simulink model "ExponentialHornDiscretized_frequencyResponse"  (Simulink 7.8)
settings: Solver=FixedStepDiscrete  StartTime=0.0  StopTime=1.0  FixedStep=1.0  RelTol=1e-3
undefined symbols (not defined in the file): areaChange, simpleDuct
settings Model: Creator=emmert  LastModifiedBy=smith

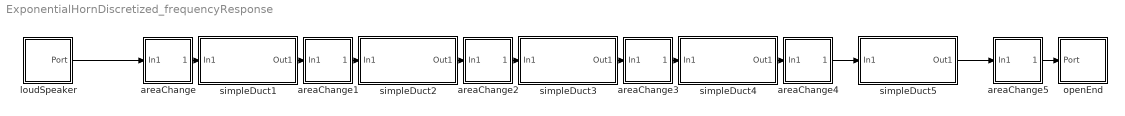
== system ExponentialHornDiscretized_frequencyResponse ==
  areaChange : Subsystem  mask{aj=1.2214}
      mask prompts: aj "Area @Out1 (m²)"
      settings: AttributesFormatString=%<aj> m^2
      mask Display:
      | plot([-.5 1.1],[.5 .5])
      | 
      | patch([ .4  .4  .3  .3  .35 .35 .15 .1 .40 .40 .10 .15 .35 .60 .60 .75 .60 .60 .75 .65 .65 .6   .6 ], ...
      |       [-.05 .05 .05 .15 .2  .25 .3 .35 .35 .65 .65 .70 .75 .75 .65 .65 .55 .45 .35 .35 .05 .05 -.05], [.85 .85 .85])
      | plot([.40 .40 .10 .15 .35 .60 .60 .75 .60 .60], ...
      |      [.35 .65 .65 .70 .75 .75 .65 .65 .55 .40])
      | plot([.1  .45 .45 .3  .3  .35 .35 .15 .1 ], ...
      |      [.35 .35 .05 .05 .15 .2  .25 .3  .35])
      | plot([.55 .6  .6  .75 .65 .65 .55 .55], ...
      |      [.35 .35 .45 .35 .35 .05 .05 .35])
      | plot([.4   .4   .6  .6 ], ...
      |      [.05 -.2 -.2   .05])
      | plot([.4   .4   .6  .6 ], ...
      |      [.05 -.2 -.2   .05])
      | 
      | text(.8,.85,'A','HorizontalAlignment','center')
  areaChange1 : Subsystem  mask{aj=1.8221}
      mask prompts: aj "Area @Out1 (m²)"
      settings: AttributesFormatString=%<aj> m^2
      mask Display:
      | plot([-.5 1.1],[.5 .5])
      | 
      | patch([ .4  .4  .3  .3  .35 .35 .15 .1 .40 .40 .10 .15 .35 .60 .60 .75 .60 .60 .75 .65 .65 .6   .6 ], ...
      |       [-.05 .05 .05 .15 .2  .25 .3 .35 .35 .65 .65 .70 .75 .75 .65 .65 .55 .45 .35 .35 .05 .05 -.05], [.85 .85 .85])
      | plot([.40 .40 .10 .15 .35 .60 .60 .75 .60 .60], ...
      |      [.35 .65 .65 .70 .75 .75 .65 .65 .55 .40])
      | plot([.1  .45 .45 .3  .3  .35 .35 .15 .1 ], ...
      |      [.35 .35 .05 .05 .15 .2  .25 .3  .35])
      | plot([.55 .6  .6  .75 .65 .65 .55 .55], ...
      |      [.35 .35 .45 .35 .35 .05 .05 .35])
      | plot([.4   .4   .6  .6 ], ...
      |      [.05 -.2 -.2   .05])
      | plot([.4   .4   .6  .6 ], ...
      |      [.05 -.2 -.2   .05])
      | 
      | text(.8,.85,'A','HorizontalAlignment','center')
  areaChange2 : Subsystem  mask{aj=2.7183}
      mask prompts: aj "Area @Out1 (m²)"
      settings: AttributesFormatString=%<aj> m^2
      mask Display:
      | plot([-.5 1.1],[.5 .5])
      | 
      | patch([ .4  .4  .3  .3  .35 .35 .15 .1 .40 .40 .10 .15 .35 .60 .60 .75 .60 .60 .75 .65 .65 .6   .6 ], ...
      |       [-.05 .05 .05 .15 .2  .25 .3 .35 .35 .65 .65 .70 .75 .75 .65 .65 .55 .45 .35 .35 .05 .05 -.05], [.85 .85 .85])
      | plot([.40 .40 .10 .15 .35 .60 .60 .75 .60 .60], ...
      |      [.35 .65 .65 .70 .75 .75 .65 .65 .55 .40])
      | plot([.1  .45 .45 .3  .3  .35 .35 .15 .1 ], ...
      |      [.35 .35 .05 .05 .15 .2  .25 .3  .35])
      | plot([.55 .6  .6  .75 .65 .65 .55 .55], ...
      |      [.35 .35 .45 .35 .35 .05 .05 .35])
      | plot([.4   .4   .6  .6 ], ...
      |      [.05 -.2 -.2   .05])
      | plot([.4   .4   .6  .6 ], ...
      |      [.05 -.2 -.2   .05])
      | 
      | text(.8,.85,'A','HorizontalAlignment','center')
  areaChange3 : Subsystem  mask{aj=4.0552}
      mask prompts: aj "Area @Out1 (m²)"
      settings: AttributesFormatString=%<aj> m^2
      mask Display:
      | plot([-.5 1.1],[.5 .5])
      | 
      | patch([ .4  .4  .3  .3  .35 .35 .15 .1 .40 .40 .10 .15 .35 .60 .60 .75 .60 .60 .75 .65 .65 .6   .6 ], ...
      |       [-.05 .05 .05 .15 .2  .25 .3 .35 .35 .65 .65 .70 .75 .75 .65 .65 .55 .45 .35 .35 .05 .05 -.05], [.85 .85 .85])
      | plot([.40 .40 .10 .15 .35 .60 .60 .75 .60 .60], ...
      |      [.35 .65 .65 .70 .75 .75 .65 .65 .55 .40])
      | plot([.1  .45 .45 .3  .3  .35 .35 .15 .1 ], ...
      |      [.35 .35 .05 .05 .15 .2  .25 .3  .35])
      | plot([.55 .6  .6  .75 .65 .65 .55 .55], ...
      |      [.35 .35 .45 .35 .35 .05 .05 .35])
      | plot([.4   .4   .6  .6 ], ...
      |      [.05 -.2 -.2   .05])
      | plot([.4   .4   .6  .6 ], ...
      |      [.05 -.2 -.2   .05])
      | 
      | text(.8,.85,'A','HorizontalAlignment','center')
  areaChange4 : Subsystem  mask{aj=6.0496}
      mask prompts: aj "Area @Out1 (m²)"
      settings: AttributesFormatString=%<aj> m^2
      mask Display:
      | plot([-.5 1.1],[.5 .5])
      | 
      | patch([ .4  .4  .3  .3  .35 .35 .15 .1 .40 .40 .10 .15 .35 .60 .60 .75 .60 .60 .75 .65 .65 .6   .6 ], ...
      |       [-.05 .05 .05 .15 .2  .25 .3 .35 .35 .65 .65 .70 .75 .75 .65 .65 .55 .45 .35 .35 .05 .05 -.05], [.85 .85 .85])
      | plot([.40 .40 .10 .15 .35 .60 .60 .75 .60 .60], ...
      |      [.35 .65 .65 .70 .75 .75 .65 .65 .55 .40])
      | plot([.1  .45 .45 .3  .3  .35 .35 .15 .1 ], ...
      |      [.35 .35 .05 .05 .15 .2  .25 .3  .35])
      | plot([.55 .6  .6  .75 .65 .65 .55 .55], ...
      |      [.35 .35 .45 .35 .35 .05 .05 .35])
      | plot([.4   .4   .6  .6 ], ...
      |      [.05 -.2 -.2   .05])
      | plot([.4   .4   .6  .6 ], ...
      |      [.05 -.2 -.2   .05])
      | 
      | text(.8,.85,'A','HorizontalAlignment','center')
  areaChange5 : Subsystem  mask{aj=7.3891}
      mask prompts: aj "Area @Out1 (m²)"
      settings: AttributesFormatString=%<aj> m^2
      mask Display:
      | plot([-.5 1.1],[.5 .5])
      | 
      | patch([ .4  .4  .3  .3  .35 .35 .15 .1 .40 .40 .10 .15 .35 .60 .60 .75 .60 .60 .75 .65 .65 .6   .6 ], ...
      |       [-.05 .05 .05 .15 .2  .25 .3 .35 .35 .65 .65 .70 .75 .75 .65 .65 .55 .45 .35 .35 .05 .05 -.05], [.85 .85 .85])
      | plot([.40 .40 .10 .15 .35 .60 .60 .75 .60 .60], ...
      |      [.35 .65 .65 .70 .75 .75 .65 .65 .55 .40])
      | plot([.1  .45 .45 .3  .3  .35 .35 .15 .1 ], ...
      |      [.35 .35 .05 .05 .15 .2  .25 .3  .35])
      | plot([.55 .6  .6  .75 .65 .65 .55 .55], ...
      |      [.35 .35 .45 .35 .35 .05 .05 .35])
      | plot([.4   .4   .6  .6 ], ...
      |      [.05 -.2 -.2   .05])
      | plot([.4   .4   .6  .6 ], ...
      |      [.05 -.2 -.2   .05])
      | 
      | text(.8,.85,'A','HorizontalAlignment','center')
  loudSpeaker : Subsystem  mask{loc=Upstream, Amp=1, c=100, Mach=0, rho=1.2, D=2*sqrt(1/pi), element=loudSpeaker}
      mask prompts: loc "Location"; Amp "Foringamplitude [m/s]"; c "Speed of sound (m/s)"; Mach "Mach number (dimensionless)"; rho "Density (Kg/m³)"; D "Diameter (m)"
      mask init:
      | if Mach<0
      |    errordlg('Mach Number must be bigger than or equal to zero','invalid Mach Number');
      | end
      | 
      | 
      | if c<=0
      |     errordlg('speed of sound must be positive','invalid speed of sound');
      | end
      | 
      | 
      | if D<=0
      |      errordlg('diameter must be positive','invalid diameter');
      | 
      | end
      | 
      | 
      | if rho<=0
      |      errordlg('density must be positive','invalid density');
      | end
      | 
      | % Set identifier
      | set_param(gcb,'element',char('loudSpeaker'));
      | 
      | switchBCUpDownStream(gcb,loc);
      mask StyleString: popup(Downstream|Upstream),edit,edit,edit,edit,edit,edit
      mask Display:
      | plot([.2 .2 .4 .4 .2],[.6 .4 .4 .6 .6])
      | plot([.7 .7 .4 .4 .7],[.9 .1 .3 .7 .9])
  openEnd : Subsystem  mask{loc=Downstream, c=343, Mach=0.1, rho=1.2, D=1, element=openEnd}
      mask prompts: loc "Location"; c "Speed of sound (m/s)"; Mach "Mach number (dimensionless)"; rho "Density (Kg/m³)"; D "Diameter (m)"
      mask init:
      | if Mach<0
      |    errordlg('Mach Number must be bigger than or equal to zero','invalid Mach Number');
      | end
      | 
      | 
      | if c<=0
      |     errordlg('speed of sound must be positive','invalid speed of sound');
      | end
      | 
      | 
      | if D<=0
      |      errordlg('diameter must be positive','invalid diameter');
      | 
      | end
      | 
      | 
      | if rho<=0
      |      errordlg('density must be positive','invalid density');
      | end
      | 
      | % Set identifier
      | set_param(gcb,'element',char('openEnd'));
      | 
      | switchBCUpDownStream(gcb,loc);
      mask StyleString: popup(Downstream|Upstream),edit,edit,edit,edit,edit
      mask Display:
      | patch([.2  1  1 .2],[.2 .2 .8 .8],[.7 1 1])
      | patch([.2 .3 .3 .2],[.2 .2 .8 .8],[.9 1 1])
      | patch([.3 .4 .4 .3],[.2 .2 .8 .8],[.8 1 1])
      | plot([.3 1],[.2 .2])
      | plot([.3 1],[.8 .8])
      | plot([1 1 0 0 1],[1 0 0 1 1])
  simpleDuct1 : Subsystem  mask{l=0.2, damping_model_popup=no damping, gm=1.4, nu=1.568e-5, Pr=0.707, damping_model_id=1}
      mask prompts: l "Length [m]"; damping_model_popup "Damping model"; gm "Ratio of specific heats [-]"; nu "Kinematic Viscosity [m^2/s]"; Pr "Prandtl number [-]"; damping_model_id "damping"
      settings: AttributesFormatString=%<l> m
      mask StyleString: edit,popup(no damping|Kirchhoff (wide tubes)|Peters|Dokumanci (best but slow)|Howe (turbulent)),edit,edit,edit,edit
      mask CallbackString:
      | |% Get the mask parameter values. This is a cell
      | %   array of strings.
      | maskStr = get_param(gcb,'MaskValues');
      | 
      | % The pop-up menu is the first mask parameter.
      | %   Check pop-up choice by comparing first letter, i.e. n or K...
      | if strcmp(maskStr{2}(1),'n'),
      |     % Turn off visibility of gamma/nu/Pr
      |     set_param(gcb,'MaskVisibilities',{'on';'on';'off';'off';'off';'off'}),
      | 	maskStr{6} = '1';
      |     set_param(gcb,'MaskValues',maskStr);
      | elseif strcmp(maskStr{2}(1),'K'),
      | 	% turn on visibility of gamma/nu/Pr
      |     set_param(gcb,'MaskVisibilities',{'on';'on';'on';'on';'on';'off'}),
      | 	maskStr{6} = '2';
      |     set_param(gcb,'MaskValues',maskStr);
      | elseif strcmp(maskStr{2}(1),'P'),
      | 	% turn on visibility of gamma/nu/Pr
      |     set_param(gcb,'MaskVisibilities',{'on';'on';'on';'on';'on';'off'}),
      | 	maskStr{6} = '3';
      |     set_param(gcb,'MaskValues',maskStr);
      | elseif strcmp(maskStr{2}(1),'D'),
      | 	% turn on visibility of gamma/nu/Pr
      |     set_param(gcb,'MaskVisibilities',{'on';'on';'on';'on';'on';'off'}),
      | 	maskStr{6} = '4';
      |     set_param(gcb,'MaskValues',maskStr);
      | else
      | 	% turn on visibility of gamma/nu
      |     set_param(gcb,'MaskVisibilities',{'on';'on';'on';'on';'off';'off'}),
      | 	maskStr{6} = '5';
      |     set_param(gcb,'MaskValues',maskStr);
      | end||||
      mask Display:
      | patch([0 1 1 0],[.2 .2 .8 .8],[.7 1 1])
      | plot([0 1],[.2 .2])
      | plot([0 1],[.8 .8])
      | 
      | plot([1 1 0 0 1],[1 0 0 1 1])
  simpleDuct2 : Subsystem  mask{l=0.2, damping_model_popup=no damping, gm=1.4, nu=1.568e-5, Pr=0.707, damping_model_id=1}
      mask prompts: l "Length [m]"; damping_model_popup "Damping model"; gm "Ratio of specific heats [-]"; nu "Kinematic Viscosity [m^2/s]"; Pr "Prandtl number [-]"; damping_model_id "damping"
      settings: AttributesFormatString=%<l> m
      mask StyleString: edit,popup(no damping|Kirchhoff (wide tubes)|Peters|Dokumanci (best but slow)|Howe (turbulent)),edit,edit,edit,edit
      mask CallbackString:
      | |% Get the mask parameter values. This is a cell
      | %   array of strings.
      | maskStr = get_param(gcb,'MaskValues');
      | 
      | % The pop-up menu is the first mask parameter.
      | %   Check pop-up choice by comparing first letter, i.e. n or K...
      | if strcmp(maskStr{2}(1),'n'),
      |     % Turn off visibility of gamma/nu/Pr
      |     set_param(gcb,'MaskVisibilities',{'on';'on';'off';'off';'off';'off'}),
      | 	maskStr{6} = '1';
      |     set_param(gcb,'MaskValues',maskStr);
      | elseif strcmp(maskStr{2}(1),'K'),
      | 	% turn on visibility of gamma/nu/Pr
      |     set_param(gcb,'MaskVisibilities',{'on';'on';'on';'on';'on';'off'}),
      | 	maskStr{6} = '2';
      |     set_param(gcb,'MaskValues',maskStr);
      | elseif strcmp(maskStr{2}(1),'P'),
      | 	% turn on visibility of gamma/nu/Pr
      |     set_param(gcb,'MaskVisibilities',{'on';'on';'on';'on';'on';'off'}),
      | 	maskStr{6} = '3';
      |     set_param(gcb,'MaskValues',maskStr);
      | elseif strcmp(maskStr{2}(1),'D'),
      | 	% turn on visibility of gamma/nu/Pr
      |     set_param(gcb,'MaskVisibilities',{'on';'on';'on';'on';'on';'off'}),
      | 	maskStr{6} = '4';
      |     set_param(gcb,'MaskValues',maskStr);
      | else
      | 	% turn on visibility of gamma/nu
      |     set_param(gcb,'MaskVisibilities',{'on';'on';'on';'on';'off';'off'}),
      | 	maskStr{6} = '5';
      |     set_param(gcb,'MaskValues',maskStr);
      | end||||
      mask Display:
      | patch([0 1 1 0],[.2 .2 .8 .8],[.7 1 1])
      | plot([0 1],[.2 .2])
      | plot([0 1],[.8 .8])
      | 
      | plot([1 1 0 0 1],[1 0 0 1 1])
  simpleDuct3 : Subsystem  mask{l=0.2, damping_model_popup=no damping, gm=1.4, nu=1.568e-5, Pr=0.707, damping_model_id=1}
      mask prompts: l "Length [m]"; damping_model_popup "Damping model"; gm "Ratio of specific heats [-]"; nu "Kinematic Viscosity [m^2/s]"; Pr "Prandtl number [-]"; damping_model_id "damping"
      settings: AttributesFormatString=%<l> m
      mask StyleString: edit,popup(no damping|Kirchhoff (wide tubes)|Peters|Dokumanci (best but slow)|Howe (turbulent)),edit,edit,edit,edit
      mask CallbackString:
      | |% Get the mask parameter values. This is a cell
      | %   array of strings.
      | maskStr = get_param(gcb,'MaskValues');
      | 
      | % The pop-up menu is the first mask parameter.
      | %   Check pop-up choice by comparing first letter, i.e. n or K...
      | if strcmp(maskStr{2}(1),'n'),
      |     % Turn off visibility of gamma/nu/Pr
      |     set_param(gcb,'MaskVisibilities',{'on';'on';'off';'off';'off';'off'}),
      | 	maskStr{6} = '1';
      |     set_param(gcb,'MaskValues',maskStr);
      | elseif strcmp(maskStr{2}(1),'K'),
      | 	% turn on visibility of gamma/nu/Pr
      |     set_param(gcb,'MaskVisibilities',{'on';'on';'on';'on';'on';'off'}),
      | 	maskStr{6} = '2';
      |     set_param(gcb,'MaskValues',maskStr);
      | elseif strcmp(maskStr{2}(1),'P'),
      | 	% turn on visibility of gamma/nu/Pr
      |     set_param(gcb,'MaskVisibilities',{'on';'on';'on';'on';'on';'off'}),
      | 	maskStr{6} = '3';
      |     set_param(gcb,'MaskValues',maskStr);
      | elseif strcmp(maskStr{2}(1),'D'),
      | 	% turn on visibility of gamma/nu/Pr
      |     set_param(gcb,'MaskVisibilities',{'on';'on';'on';'on';'on';'off'}),
      | 	maskStr{6} = '4';
      |     set_param(gcb,'MaskValues',maskStr);
      | else
      | 	% turn on visibility of gamma/nu
      |     set_param(gcb,'MaskVisibilities',{'on';'on';'on';'on';'off';'off'}),
      | 	maskStr{6} = '5';
      |     set_param(gcb,'MaskValues',maskStr);
      | end||||
      mask Display:
      | patch([0 1 1 0],[.2 .2 .8 .8],[.7 1 1])
      | plot([0 1],[.2 .2])
      | plot([0 1],[.8 .8])
      | 
      | plot([1 1 0 0 1],[1 0 0 1 1])
  simpleDuct4 : Subsystem  mask{l=0.2, damping_model_popup=no damping, gm=1.4, nu=1.568e-5, Pr=0.707, damping_model_id=1}
      mask prompts: l "Length [m]"; damping_model_popup "Damping model"; gm "Ratio of specific heats [-]"; nu "Kinematic Viscosity [m^2/s]"; Pr "Prandtl number [-]"; damping_model_id "damping"
      settings: AttributesFormatString=%<l> m
      mask StyleString: edit,popup(no damping|Kirchhoff (wide tubes)|Peters|Dokumanci (best but slow)|Howe (turbulent)),edit,edit,edit,edit
      mask CallbackString:
      | |% Get the mask parameter values. This is a cell
      | %   array of strings.
      | maskStr = get_param(gcb,'MaskValues');
      | 
      | % The pop-up menu is the first mask parameter.
      | %   Check pop-up choice by comparing first letter, i.e. n or K...
      | if strcmp(maskStr{2}(1),'n'),
      |     % Turn off visibility of gamma/nu/Pr
      |     set_param(gcb,'MaskVisibilities',{'on';'on';'off';'off';'off';'off'}),
      | 	maskStr{6} = '1';
      |     set_param(gcb,'MaskValues',maskStr);
      | elseif strcmp(maskStr{2}(1),'K'),
      | 	% turn on visibility of gamma/nu/Pr
      |     set_param(gcb,'MaskVisibilities',{'on';'on';'on';'on';'on';'off'}),
      | 	maskStr{6} = '2';
      |     set_param(gcb,'MaskValues',maskStr);
      | elseif strcmp(maskStr{2}(1),'P'),
      | 	% turn on visibility of gamma/nu/Pr
      |     set_param(gcb,'MaskVisibilities',{'on';'on';'on';'on';'on';'off'}),
      | 	maskStr{6} = '3';
      |     set_param(gcb,'MaskValues',maskStr);
      | elseif strcmp(maskStr{2}(1),'D'),
      | 	% turn on visibility of gamma/nu/Pr
      |     set_param(gcb,'MaskVisibilities',{'on';'on';'on';'on';'on';'off'}),
      | 	maskStr{6} = '4';
      |     set_param(gcb,'MaskValues',maskStr);
      | else
      | 	% turn on visibility of gamma/nu
      |     set_param(gcb,'MaskVisibilities',{'on';'on';'on';'on';'off';'off'}),
      | 	maskStr{6} = '5';
      |     set_param(gcb,'MaskValues',maskStr);
      | end||||
      mask Display:
      | patch([0 1 1 0],[.2 .2 .8 .8],[.7 1 1])
      | plot([0 1],[.2 .2])
      | plot([0 1],[.8 .8])
      | 
      | plot([1 1 0 0 1],[1 0 0 1 1])
  simpleDuct5 : Subsystem  mask{l=0.2, damping_model_popup=no damping, gm=1.4, nu=1.568e-5, Pr=0.707, damping_model_id=1}
      mask prompts: l "Length [m]"; damping_model_popup "Damping model"; gm "Ratio of specific heats [-]"; nu "Kinematic Viscosity [m^2/s]"; Pr "Prandtl number [-]"; damping_model_id "damping"
      settings: AttributesFormatString=%<l> m
      mask StyleString: edit,popup(no damping|Kirchhoff (wide tubes)|Peters|Dokumanci (best but slow)|Howe (turbulent)),edit,edit,edit,edit
      mask CallbackString:
      | |% Get the mask parameter values. This is a cell
      | %   array of strings.
      | maskStr = get_param(gcb,'MaskValues');
      | 
      | % The pop-up menu is the first mask parameter.
      | %   Check pop-up choice by comparing first letter, i.e. n or K...
      | if strcmp(maskStr{2}(1),'n'),
      |     % Turn off visibility of gamma/nu/Pr
      |     set_param(gcb,'MaskVisibilities',{'on';'on';'off';'off';'off';'off'}),
      | 	maskStr{6} = '1';
      |     set_param(gcb,'MaskValues',maskStr);
      | elseif strcmp(maskStr{2}(1),'K'),
      | 	% turn on visibility of gamma/nu/Pr
      |     set_param(gcb,'MaskVisibilities',{'on';'on';'on';'on';'on';'off'}),
      | 	maskStr{6} = '2';
      |     set_param(gcb,'MaskValues',maskStr);
      | elseif strcmp(maskStr{2}(1),'P'),
      | 	% turn on visibility of gamma/nu/Pr
      |     set_param(gcb,'MaskVisibilities',{'on';'on';'on';'on';'on';'off'}),
      | 	maskStr{6} = '3';
      |     set_param(gcb,'MaskValues',maskStr);
      | elseif strcmp(maskStr{2}(1),'D'),
      | 	% turn on visibility of gamma/nu/Pr
      |     set_param(gcb,'MaskVisibilities',{'on';'on';'on';'on';'on';'off'}),
      | 	maskStr{6} = '4';
      |     set_param(gcb,'MaskValues',maskStr);
      | else
      | 	% turn on visibility of gamma/nu
      |     set_param(gcb,'MaskVisibilities',{'on';'on';'on';'on';'off';'off'}),
      | 	maskStr{6} = '5';
      |     set_param(gcb,'MaskValues',maskStr);
      | end||||
      mask Display:
      | patch([0 1 1 0],[.2 .2 .8 .8],[.7 1 1])
      | plot([0 1],[.2 .2])
      | plot([0 1],[.8 .8])
      | 
      | plot([1 1 0 0 1],[1 0 0 1 1])
  wires:
  loudSpeaker/1(Port) -> areaChange/1(In1)
  areaChange/1(Out1) -> simpleDuct1/1(In1)
  simpleDuct1/1(Out1) -> areaChange1/1(In1)
  areaChange1/1(Out1) -> simpleDuct2/1(In1)
  simpleDuct2/1(Out1) -> areaChange2/1(In1)
  areaChange2/1(Out1) -> simpleDuct3/1(In1)
  simpleDuct3/1(Out1) -> areaChange3/1(In1)
  areaChange3/1(Out1) -> simpleDuct4/1(In1)
  simpleDuct4/1(Out1) -> areaChange4/1(In1)
  areaChange4/1(Out1) -> simpleDuct5/1(In1)
  simpleDuct5/1(Out1) -> areaChange5/1(In1)
  areaChange5/1(Out1) -> openEnd/1(Port)

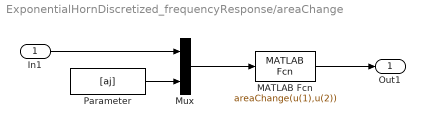
== system ExponentialHornDiscretized_frequencyResponse/areaChange ==
  In1 : Inport
  MATLAB Fcn : MATLABFcn  MATLABFcn=areaChange(u(1),u(2))  OutputDimensions=1  OutputSignalType=real
  Mux : Mux  Inputs=2
  Parameter : Constant  Value=[aj]
  Out1 : Outport
  wires:
  Parameter/1 -> Mux/2
  Mux/1 -> MATLAB Fcn/1
  MATLAB Fcn/1 -> Out1/1
  In1/1 -> Mux/1

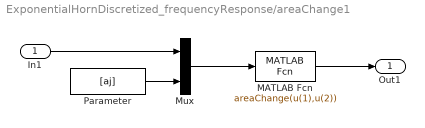
== system ExponentialHornDiscretized_frequencyResponse/areaChange1 ==
  In1 : Inport
  MATLAB Fcn : MATLABFcn  MATLABFcn=areaChange(u(1),u(2))  OutputDimensions=1  OutputSignalType=real
  Mux : Mux  Inputs=2
  Parameter : Constant  Value=[aj]
  Out1 : Outport
  wires:
  Parameter/1 -> Mux/2
  Mux/1 -> MATLAB Fcn/1
  MATLAB Fcn/1 -> Out1/1
  In1/1 -> Mux/1

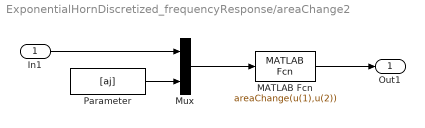
== system ExponentialHornDiscretized_frequencyResponse/areaChange2 ==
  In1 : Inport
  MATLAB Fcn : MATLABFcn  MATLABFcn=areaChange(u(1),u(2))  OutputDimensions=1  OutputSignalType=real
  Mux : Mux  Inputs=2
  Parameter : Constant  Value=[aj]
  Out1 : Outport
  wires:
  Parameter/1 -> Mux/2
  Mux/1 -> MATLAB Fcn/1
  MATLAB Fcn/1 -> Out1/1
  In1/1 -> Mux/1

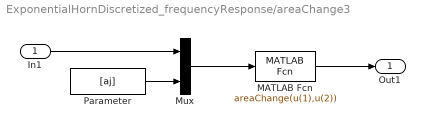
== system ExponentialHornDiscretized_frequencyResponse/areaChange3 ==
  In1 : Inport
  MATLAB Fcn : MATLABFcn  MATLABFcn=areaChange(u(1),u(2))  OutputDimensions=1  OutputSignalType=real
  Mux : Mux  Inputs=2
  Parameter : Constant  Value=[aj]
  Out1 : Outport
  wires:
  Parameter/1 -> Mux/2
  Mux/1 -> MATLAB Fcn/1
  MATLAB Fcn/1 -> Out1/1
  In1/1 -> Mux/1

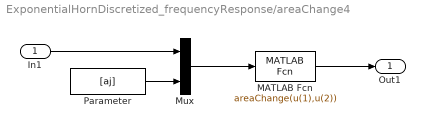
== system ExponentialHornDiscretized_frequencyResponse/areaChange4 ==
  In1 : Inport
  MATLAB Fcn : MATLABFcn  MATLABFcn=areaChange(u(1),u(2))  OutputDimensions=1  OutputSignalType=real
  Mux : Mux  Inputs=2
  Parameter : Constant  Value=[aj]
  Out1 : Outport
  wires:
  Parameter/1 -> Mux/2
  Mux/1 -> MATLAB Fcn/1
  MATLAB Fcn/1 -> Out1/1
  In1/1 -> Mux/1

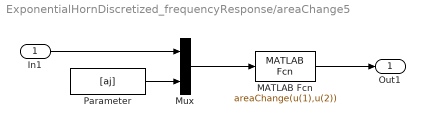
== system ExponentialHornDiscretized_frequencyResponse/areaChange5 ==
  In1 : Inport
  MATLAB Fcn : MATLABFcn  MATLABFcn=areaChange(u(1),u(2))  OutputDimensions=1  OutputSignalType=real
  Mux : Mux  Inputs=2
  Parameter : Constant  Value=[aj]
  Out1 : Outport
  wires:
  Parameter/1 -> Mux/2
  Mux/1 -> MATLAB Fcn/1
  MATLAB Fcn/1 -> Out1/1
  In1/1 -> Mux/1

== system ExponentialHornDiscretized_frequencyResponse/loudSpeaker ==
  Port : Outport

== system ExponentialHornDiscretized_frequencyResponse/openEnd ==
  Port : Inport

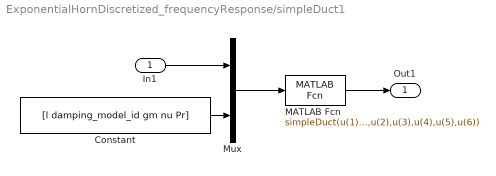
== system ExponentialHornDiscretized_frequencyResponse/simpleDuct1 ==
  In1 : Inport
  Constant : Constant  Value=[l damping_model_id gm nu Pr]
  MATLAB Fcn : MATLABFcn  MATLABFcn=simpleDuct(u(1),u(2),u(3),u(4),u(5),u(6))
  Mux : Mux  Inputs=2
  Out1 : Outport
  wires:
  In1/1 -> Mux/1
  Mux/1 -> MATLAB Fcn/1
  MATLAB Fcn/1 -> Out1/1
  Constant/1 -> Mux/2

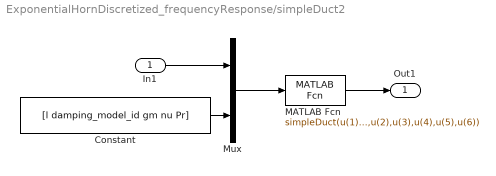
== system ExponentialHornDiscretized_frequencyResponse/simpleDuct2 ==
  In1 : Inport
  Constant : Constant  Value=[l damping_model_id gm nu Pr]
  MATLAB Fcn : MATLABFcn  MATLABFcn=simpleDuct(u(1),u(2),u(3),u(4),u(5),u(6))
  Mux : Mux  Inputs=2
  Out1 : Outport
  wires:
  In1/1 -> Mux/1
  Mux/1 -> MATLAB Fcn/1
  MATLAB Fcn/1 -> Out1/1
  Constant/1 -> Mux/2

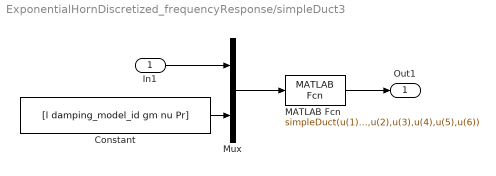
== system ExponentialHornDiscretized_frequencyResponse/simpleDuct3 ==
  In1 : Inport
  Constant : Constant  Value=[l damping_model_id gm nu Pr]
  MATLAB Fcn : MATLABFcn  MATLABFcn=simpleDuct(u(1),u(2),u(3),u(4),u(5),u(6))
  Mux : Mux  Inputs=2
  Out1 : Outport
  wires:
  In1/1 -> Mux/1
  Mux/1 -> MATLAB Fcn/1
  MATLAB Fcn/1 -> Out1/1
  Constant/1 -> Mux/2

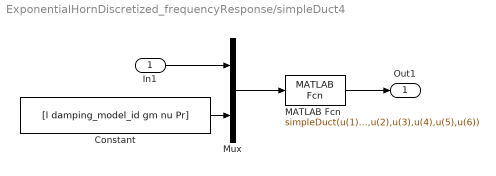
== system ExponentialHornDiscretized_frequencyResponse/simpleDuct4 ==
  In1 : Inport
  Constant : Constant  Value=[l damping_model_id gm nu Pr]
  MATLAB Fcn : MATLABFcn  MATLABFcn=simpleDuct(u(1),u(2),u(3),u(4),u(5),u(6))
  Mux : Mux  Inputs=2
  Out1 : Outport
  wires:
  In1/1 -> Mux/1
  Mux/1 -> MATLAB Fcn/1
  MATLAB Fcn/1 -> Out1/1
  Constant/1 -> Mux/2

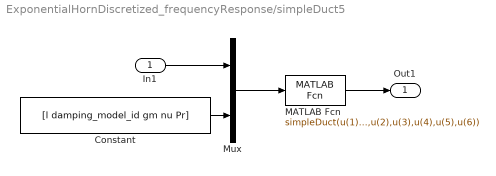
== system ExponentialHornDiscretized_frequencyResponse/simpleDuct5 ==
  In1 : Inport
  Constant : Constant  Value=[l damping_model_id gm nu Pr]
  MATLAB Fcn : MATLABFcn  MATLABFcn=simpleDuct(u(1),u(2),u(3),u(4),u(5),u(6))
  Mux : Mux  Inputs=2
  Out1 : Outport
  wires:
  In1/1 -> Mux/1
  Mux/1 -> MATLAB Fcn/1
  MATLAB Fcn/1 -> Out1/1
  Constant/1 -> Mux/2
